simulink model "quad_control"  (Simulink 10.0)
settings: Solver=ode45  StartTime=0.0  StopTime=20  RelTol=1e-3  EnableMultiTasking=on
undefined symbols (not defined in the file): X, x, Y, Z
libraries: sm_lib x84, nesl_utility x46, simulink x30, fl_lib x4, sm_double_wishbone_suspension_lib x2, aerolibtransform2 x2, vrlib x1
(part 3 of 3)

== system quad_control/Controlled Quadrotor2/Quad and sensors/Quad_base_frame ==
  ReferenceFrame : sm_lib/Frames and  Transforms/Reference  Frame  BlockFunction=simmechanics.library.frames_transforms.reference_frame
      settings: SourceProductName=Simscape Multibody  SourceProductBaseCode=MS
  Solid : sm_lib/Body Elements/Solid  InertiaType=Custom  Mass=0.08666672774597016  MassUnits=kg  CenterOfMass=[0 0 0]  CenterOfMassUnits=cm  MomentsOfInertia=[2.1975971956009444 4.1375830610397539 2.1893109381556854]  MomentsOfInertiaUnits=kg*cm^2  ProductsOfInertia=[0 0 0]  ProductsOfInertiaUnits=kg*cm^2  DensityBased=on  Density=1000  DensityUnits=kg/(m^3)  GraphicType=FromGeometry  MarkerShape=Sphere  MarkerSize=10  MarkerSizeUnits=m  GraphicVisPropType=SimpleVisualProperties  GraphicDiffuseColor=[1.0 1.0 0.0]  GraphicSpecularColor=[0.5 0.5 0.5 1.0]  GraphicAmbientColor=[0.15 0.15 0.15 1.0]  GraphicEmissiveColor=[0.0 0.0 0.0 1.0]  GraphicShininess=75  GraphicOpacity=1  GeometryShape=FromFile  RectangleSize=[1 1]  RectangleSizeUnits=m  BrickDimensions=[1 1 1]  BrickDimensionUnits=m  CylinderRadius=1  CylinderRadiusUnits=m  CylinderLength=1  CylinderLengthUnits=m  SphereRadius=1  SphereRadiusUnits=m  EllipsoidRadii=[1 1 1]  EllipsoidRadiiUnits=m  ExtrusionCrossSection=[1 1; -1 1; -1 -1; 1 -1]  ExtrusionCrossSectionUnits=m  ExtrusionLength=1  ExtrusionLengthUnits=m  PolygonNumSides=3  PolygonOuterRadius=1  PolygonOuterRadiusUnits=m  ExtGeomFileType=STL  ExtGeomFileName=frame_motors_prt_Default_sldprt.STL  ExtGeomFileUnits=cm  RevolutionCrossSection=[1 1; 1 -1; 2 -1; 2 1]  RevolutionCrossSectionUnits=m  RevolutionExtent=Full  RevolutionAngle=180  RevolutionAngleUnits=deg  BlockFunction=simmechanics.library.body_elements.solid
  Transform : sm_lib/Frames and  Transforms/Rigid  Transform  TranslationMethod=Cartesian  TranslationLengthUnit=cm  TranslationStandardAxis=+Z  TranslationStandardOffset=0  TranslationCartesianOffset=[0.0025633413850464047 11.008725718944405 2.3329463666203418]  TranslationROffset=0  TranslationROffsetUnits=m  TranslationZOffset=0  TranslationZOffsetUnits=m  TranslationThetaOffset=0  TranslationThetaOffsetUnits=deg  RotationMethod=ArbitraryAxis  RotationAngleUnits=rad  RotationStandardAxis=+Z  RotationAngle=3.1415926535897896  RotationArbitraryAxis=[-1 -0 -0]  FollAlignAxisA=+X  BaseAlignAxisA=+Y  FollAlignAxisB=+Y  BaseAlignAxisB=+Z  RotationMatrix=[1 0 0; 0 1 0; 0 0 1]  BlockFunction=simmechanics.library.frames_transforms.rigid_transform
      settings: SourceProductName=Simscape Multibody  SourceProductBaseCode=MS
  Transform1 : sm_lib/Frames and  Transforms/Rigid  Transform  TranslationMethod=Cartesian  TranslationLengthUnit=cm  TranslationStandardAxis=+Z  TranslationStandardOffset=0  TranslationCartesianOffset=[0.002563341385239306 -10.791274281055713 2.3329463666202659]  TranslationROffset=0  TranslationROffsetUnits=m  TranslationZOffset=0  TranslationZOffsetUnits=m  TranslationThetaOffset=0  TranslationThetaOffsetUnits=deg  RotationMethod=ArbitraryAxis  RotationAngleUnits=rad  RotationStandardAxis=+Z  RotationAngle=3.1415926535897896  RotationArbitraryAxis=[-1 -0 -0]  FollAlignAxisA=+X  BaseAlignAxisA=+Y  FollAlignAxisB=+Y  BaseAlignAxisB=+Z  RotationMatrix=[1 0 0; 0 1 0; 0 0 1]  BlockFunction=simmechanics.library.frames_transforms.rigid_transform
      settings: SourceProductName=Simscape Multibody  SourceProductBaseCode=MS
  Transform2 : sm_lib/Frames and  Transforms/Rigid  Transform  TranslationMethod=Cartesian  TranslationLengthUnit=cm  TranslationStandardAxis=+Z  TranslationStandardOffset=0  TranslationCartesianOffset=[10.902563341385184 0.10872571894443728 2.3329463666203041]  TranslationROffset=0  TranslationROffsetUnits=m  TranslationZOffset=0  TranslationZOffsetUnits=m  TranslationThetaOffset=0  TranslationThetaOffsetUnits=deg  RotationMethod=ArbitraryAxis  RotationAngleUnits=rad  RotationStandardAxis=+Z  RotationAngle=3.1415926535897896  RotationArbitraryAxis=[-1 -0 -0]  FollAlignAxisA=+X  BaseAlignAxisA=+Y  FollAlignAxisB=+Y  BaseAlignAxisB=+Z  RotationMatrix=[1 0 0; 0 1 0; 0 0 1]  BlockFunction=simmechanics.library.frames_transforms.rigid_transform
      settings: SourceProductName=Simscape Multibody  SourceProductBaseCode=MS
  Transform3 : sm_lib/Frames and  Transforms/Rigid  Transform  TranslationMethod=Cartesian  TranslationLengthUnit=cm  TranslationStandardAxis=+Z  TranslationStandardOffset=0  TranslationCartesianOffset=[-10.897436658614925 0.10872571894425409 2.3329463666203041]  TranslationROffset=0  TranslationROffsetUnits=m  TranslationZOffset=0  TranslationZOffsetUnits=m  TranslationThetaOffset=0  TranslationThetaOffsetUnits=deg  RotationMethod=ArbitraryAxis  RotationAngleUnits=rad  RotationStandardAxis=+Z  RotationAngle=3.1415926535897896  RotationArbitraryAxis=[-1 -0 -0]  FollAlignAxisA=+X  BaseAlignAxisA=+Y  FollAlignAxisB=+Y  BaseAlignAxisB=+Z  RotationMatrix=[1 0 0; 0 1 0; 0 0 1]  BlockFunction=simmechanics.library.frames_transforms.rigid_transform
      settings: SourceProductName=Simscape Multibody  SourceProductBaseCode=MS
  F4 : PMIOPort  Side=Left
  F3 : PMIOPort  Port=2  Side=Right
  F2 : PMIOPort  Port=3  Side=Right
  F1 : PMIOPort  Port=4  Side=Right
  F : PMIOPort  Port=5  Side=Right
  connections:
  Transform3/LConn1 -- F4/RConn1 -- Transform/LConn1 -- Transform1/LConn1 -- Transform2/LConn1 -- ReferenceFrame/RConn1 -- Solid/RConn1
  Transform/RConn1 -- F/RConn1
  Transform1/RConn1 -- F1/RConn1
  Transform2/RConn1 -- F2/RConn1
  Transform3/RConn1 -- F3/RConn1

== system quad_control/Controlled Quadrotor2/world_base_and_floor/Floor ==
  ReferenceFrame : sm_lib/Frames and  Transforms/Reference  Frame  BlockFunction=simmechanics.library.frames_transforms.reference_frame
      settings: SourceProductName=Simscape Multibody  SourceProductBaseCode=MS
  Solid : sm_lib/Body Elements/Solid  InertiaType=Custom  Mass=3116.2499999999991  MassUnits=kg  CenterOfMass=[-7.9936057773011283e-16 -7.6605388699135795e-16 0.049999999999999996]  CenterOfMassUnits=m  MomentsOfInertia=[6494.7843749999947 6494.7843749999965 12984.374999999993]  MomentsOfInertiaUnits=kg*m^2  ProductsOfInertia=[0 0 -1.8451906669270059e-13]  ProductsOfInertiaUnits=kg*m^2  DensityBased=on  Density=1000  DensityUnits=kg/(m^3)  GraphicType=FromGeometry  MarkerShape=Sphere  MarkerSize=10  MarkerSizeUnits=m  GraphicVisPropType=SimpleVisualProperties  GraphicDiffuseColor=[0.0 0.4 0.4]  GraphicSpecularColor=[0.5 0.5 0.5 1.0]  GraphicAmbientColor=[0.15 0.15 0.15 1.0]  GraphicEmissiveColor=[0.0 0.0 0.0 1.0]  GraphicShininess=75  GraphicOpacity=1  GeometryShape=FromFile  RectangleSize=[1 1]  RectangleSizeUnits=m  BrickDimensions=[1 1 1]  BrickDimensionUnits=m  CylinderRadius=1  CylinderRadiusUnits=m  CylinderLength=1  CylinderLengthUnits=m  SphereRadius=1  SphereRadiusUnits=m  EllipsoidRadii=[1 1 1]  EllipsoidRadiiUnits=m  ExtrusionCrossSection=[1 1; -1 1; -1 -1; 1 -1]  ExtrusionCrossSectionUnits=m  ExtrusionLength=1  ExtrusionLengthUnits=m  PolygonNumSides=3  PolygonOuterRadius=1  PolygonOuterRadiusUnits=m  ExtGeomFileType=STL  ExtGeomFileName=floor_Default_sldprt.STL  ExtGeomFileUnits=m  RevolutionCrossSection=[1 1; 1 -1; 2 -1; 2 1]  RevolutionCrossSectionUnits=m  RevolutionExtent=Full  RevolutionAngle=180  RevolutionAngleUnits=deg  BlockFunction=simmechanics.library.body_elements.solid
  F : PMIOPort  Side=Left
  connections:
  ReferenceFrame/RConn1 -- Solid/RConn1 -- F/RConn1

== system quad_control/Controlled Quadrotor2/world_base_and_floor/floor2_1_RIGID ==
  ReferenceFrame : sm_lib/Frames and  Transforms/Reference  Frame  BlockFunction=simmechanics.library.frames_transforms.reference_frame
      settings: SourceProductName=Simscape Multibody  SourceProductBaseCode=MS
  Solid : sm_lib/Body Elements/Solid  InertiaType=Custom  Mass=2385.7763976055348  MassUnits=kg  CenterOfMass=[0.0012364446490796092 -0.0050570097364130108 0.050000002292491054]  CenterOfMassUnits=m  MomentsOfInertia=[5164.4159493771613 5045.1873132107048 10205.643458365917]  MomentsOfInertiaUnits=kg*m^2  ProductsOfInertia=[-1.8888660103894037e-06 -1.1052348010530633e-05 -9.5984261339922075]  ProductsOfInertiaUnits=kg*m^2  DensityBased=on  Density=1000  DensityUnits=kg/(m^3)  GraphicType=FromGeometry  MarkerShape=Sphere  MarkerSize=10  MarkerSizeUnits=m  GraphicVisPropType=SimpleVisualProperties  GraphicDiffuseColor=[1 1 1]  GraphicSpecularColor=[0.5 0.5 0.5 1.0]  GraphicAmbientColor=[0.15 0.15 0.15 1.0]  GraphicEmissiveColor=[0.0 0.0 0.0 1.0]  GraphicShininess=75  GraphicOpacity=1  GeometryShape=FromFile  RectangleSize=[1 1]  RectangleSizeUnits=m  BrickDimensions=[1 1 1]  BrickDimensionUnits=m  CylinderRadius=1  CylinderRadiusUnits=m  CylinderLength=1  CylinderLengthUnits=m  SphereRadius=1  SphereRadiusUnits=m  EllipsoidRadii=[1 1 1]  EllipsoidRadiiUnits=m  ExtrusionCrossSection=[1 1; -1 1; -1 -1; 1 -1]  ExtrusionCrossSectionUnits=m  ExtrusionLength=1  ExtrusionLengthUnits=m  PolygonNumSides=3  PolygonOuterRadius=1  PolygonOuterRadiusUnits=m  ExtGeomFileType=STL  ExtGeomFileName=floor2_Default_sldprt.STL  ExtGeomFileUnits=m  RevolutionCrossSection=[1 1; 1 -1; 2 -1; 2 1]  RevolutionCrossSectionUnits=m  RevolutionExtent=Full  RevolutionAngle=180  RevolutionAngleUnits=deg  BlockFunction=simmechanics.library.body_elements.solid
  Transform : sm_lib/Frames and  Transforms/Rigid  Transform  TranslationMethod=Cartesian  TranslationLengthUnit=m  TranslationStandardAxis=+Z  TranslationStandardOffset=0  TranslationCartesianOffset=[0 0 0.099999999999999978]  TranslationROffset=0  TranslationROffsetUnits=m  TranslationZOffset=0  TranslationZOffsetUnits=m  TranslationThetaOffset=0  TranslationThetaOffsetUnits=deg  RotationMethod=ArbitraryAxis  RotationAngleUnits=rad  RotationStandardAxis=+Z  RotationAngle=0  RotationArbitraryAxis=[0 0 0]  FollAlignAxisA=+X  BaseAlignAxisA=+Y  FollAlignAxisB=+Y  BaseAlignAxisB=+Z  RotationMatrix=[1 0 0; 0 1 0; 0 0 1]  BlockFunction=simmechanics.library.frames_transforms.rigid_transform
      settings: SourceProductName=Simscape Multibody  SourceProductBaseCode=MS
  F1 : PMIOPort  Side=Left
  connections:
  ReferenceFrame/RConn1 -- Solid/RConn1 -- Transform/LConn1 -- F1/RConn1

== system quad_control/Controlled Quadrotor2/world_base_and_floor/text2_1_RIGID ==
  ReferenceFrame : sm_lib/Frames and  Transforms/Reference  Frame  BlockFunction=simmechanics.library.frames_transforms.reference_frame
      settings: SourceProductName=Simscape Multibody  SourceProductBaseCode=MS
  Solid : sm_lib/Body Elements/Solid  InertiaType=Custom  Mass=52.995915434963941  MassUnits=kg  CenterOfMass=[0.014313236427579184 0.013266517593960889 0.050000099576434989]  CenterOfMassUnits=m  MomentsOfInertia=[1.2121218611867071 89.98262862045047 91.106423651417629]  MomentsOfInertiaUnits=kg*m^2  ProductsOfInertia=[-2.6542355925642964e-07 -7.9011888790530038e-06 1.0815100741629544]  ProductsOfInertiaUnits=kg*m^2  DensityBased=on  Density=1000  DensityUnits=kg/(m^3)  GraphicType=FromGeometry  MarkerShape=Sphere  MarkerSize=10  MarkerSizeUnits=m  GraphicVisPropType=SimpleVisualProperties  GraphicDiffuseColor=[1.0 1.0 0.4]  GraphicSpecularColor=[0.5 0.5 0.5 1.0]  GraphicAmbientColor=[0.15 0.15 0.15 1.0]  GraphicEmissiveColor=[0.0 0.0 0.0 1.0]  GraphicShininess=75  GraphicOpacity=1  GeometryShape=FromFile  RectangleSize=[1 1]  RectangleSizeUnits=m  BrickDimensions=[1 1 1]  BrickDimensionUnits=m  CylinderRadius=1  CylinderRadiusUnits=m  CylinderLength=1  CylinderLengthUnits=m  SphereRadius=1  SphereRadiusUnits=m  EllipsoidRadii=[1 1 1]  EllipsoidRadiiUnits=m  ExtrusionCrossSection=[1 1; -1 1; -1 -1; 1 -1]  ExtrusionCrossSectionUnits=m  ExtrusionLength=1  ExtrusionLengthUnits=m  PolygonNumSides=3  PolygonOuterRadius=1  PolygonOuterRadiusUnits=m  ExtGeomFileType=STL  ExtGeomFileName=text2_Default_sldprt.STL  ExtGeomFileUnits=m  RevolutionCrossSection=[1 1; 1 -1; 2 -1; 2 1]  RevolutionCrossSectionUnits=m  RevolutionExtent=Full  RevolutionAngle=180  RevolutionAngleUnits=deg  BlockFunction=simmechanics.library.body_elements.solid
  Transform : sm_lib/Frames and  Transforms/Rigid  Transform  TranslationMethod=Cartesian  TranslationLengthUnit=m  TranslationStandardAxis=+Z  TranslationStandardOffset=0  TranslationCartesianOffset=[-0.0410033698434355 2.1287464318513987 -1.3877787807814457e-17]  TranslationROffset=0  TranslationROffsetUnits=m  TranslationZOffset=0  TranslationZOffsetUnits=m  TranslationThetaOffset=0  TranslationThetaOffsetUnits=deg  RotationMethod=ArbitraryAxis  RotationAngleUnits=rad  RotationStandardAxis=+Z  RotationAngle=0  RotationArbitraryAxis=[0 0 0]  FollAlignAxisA=+X  BaseAlignAxisA=+Y  FollAlignAxisB=+Y  BaseAlignAxisB=+Z  RotationMatrix=[1 0 0; 0 1 0; 0 0 1]  BlockFunction=simmechanics.library.frames_transforms.rigid_transform
      settings: SourceProductName=Simscape Multibody  SourceProductBaseCode=MS
  F1 : PMIOPort  Side=Left
  connections:
  Transform/LConn1 -- F1/RConn1 -- ReferenceFrame/RConn1 -- Solid/RConn1

== system quad_control/Controlled Quadrotor1/Quad and sensors/Engine1/x5x3R_Propeller_1_RIGID ==
  ReferenceFrame : sm_lib/Frames and  Transforms/Reference  Frame  BlockFunction=simmechanics.library.frames_transforms.reference_frame
      settings: SourceProductName=Simscape Multibody  SourceProductBaseCode=MS
  Solid : sm_lib/Body Elements/Solid  InertiaType=Custom  Mass=0.0016554437499046806  MassUnits=kg  CenterOfMass=[-9.4091969973109005e-06 1.1743794416735667 -1.1742585501049463]  CenterOfMassUnits=mm  MomentsOfInertia=[1.470390252449407 0.013647828129438603 1.4797649971234468]  MomentsOfInertiaUnits=kg*mm^2  ProductsOfInertia=[7.6225900321173699e-07 3.0379766986994385e-08 -0.023426386413677357]  ProductsOfInertiaUnits=kg*mm^2  DensityBased=on  Density=1000  DensityUnits=kg/(m^3)  GraphicType=FromGeometry  MarkerShape=Sphere  MarkerSize=10  MarkerSizeUnits=m  GraphicVisPropType=SimpleVisualProperties  GraphicDiffuseColor=[1.0 0.2 0.0]  GraphicSpecularColor=[0.5 0.5 0.5 1.0]  GraphicAmbientColor=[0.15 0.15 0.15 1.0]  GraphicEmissiveColor=[0.0 0.0 0.0 1.0]  GraphicShininess=75  GraphicOpacity=1  GeometryShape=FromFile  RectangleSize=[1 1]  RectangleSizeUnits=m  BrickDimensions=[1 1 1]  BrickDimensionUnits=m  CylinderRadius=1  CylinderRadiusUnits=m  CylinderLength=1  CylinderLengthUnits=m  SphereRadius=1  SphereRadiusUnits=m  EllipsoidRadii=[1 1 1]  EllipsoidRadiiUnits=m  ExtrusionCrossSection=[1 1; -1 1; -1 -1; 1 -1]  ExtrusionCrossSectionUnits=m  ExtrusionLength=1  ExtrusionLengthUnits=m  PolygonNumSides=3  PolygonOuterRadius=1  PolygonOuterRadiusUnits=m  ExtGeomFileType=STL  ExtGeomFileName=5x3R Propeller_Default_sldprt.STL  ExtGeomFileUnits=mm  RevolutionCrossSection=[1 1; 1 -1; 2 -1; 2 1]  RevolutionCrossSectionUnits=m  RevolutionExtent=Full  RevolutionAngle=180  RevolutionAngleUnits=deg  BlockFunction=simmechanics.library.body_elements.solid
  Transform : sm_lib/Frames and  Transforms/Rigid  Transform  TranslationMethod=Cartesian  TranslationLengthUnit=cm  TranslationStandardAxis=+Z  TranslationStandardOffset=0  TranslationCartesianOffset=[2.2204460492503131e-16 0.117384178389595 0.70211061015740817]  TranslationROffset=0  TranslationROffsetUnits=m  TranslationZOffset=0  TranslationZOffsetUnits=m  TranslationThetaOffset=0  TranslationThetaOffsetUnits=deg  RotationMethod=ArbitraryAxis  RotationAngleUnits=rad  RotationStandardAxis=+Z  RotationAngle=3.14159265358979  RotationArbitraryAxis=[-1 -2.9659662640582496e-31 1.7826123921481009e-16]  FollAlignAxisA=+X  BaseAlignAxisA=+Y  FollAlignAxisB=+Y  BaseAlignAxisB=+Z  RotationMatrix=[1 0 0; 0 1 0; 0 0 1]  BlockFunction=simmechanics.library.frames_transforms.rigid_transform
      settings: SourceProductName=Simscape Multibody  SourceProductBaseCode=MS
  F : PMIOPort  Side=Left
  connections:
  ReferenceFrame/RConn1 -- Solid/RConn1 -- Transform/LConn1
  Transform/RConn1 -- F/RConn1

== system quad_control/Controlled Quadrotor1/Quad and sensors/Engine2/x5x3L_Propeller_1_RIGID ==
  ReferenceFrame : sm_lib/Frames and  Transforms/Reference  Frame  BlockFunction=simmechanics.library.frames_transforms.reference_frame
      settings: SourceProductName=Simscape Multibody  SourceProductBaseCode=MS
  Solid : sm_lib/Body Elements/Solid  InertiaType=Custom  Mass=0.0016554447827057072  MassUnits=kg  CenterOfMass=[-1.7940684369643517e-05 0.00054453975800766252 -0.0036928877456850299]  CenterOfMassUnits=mm  MomentsOfInertia=[1.4703904309245746 0.013647735813102926 1.4797650826066844]  MomentsOfInertiaUnits=kg*mm^2  ProductsOfInertia=[7.6907097391567737e-07 1.5969591997949786e-08 -0.023426501249338923]  ProductsOfInertiaUnits=kg*mm^2  DensityBased=on  Density=1000  DensityUnits=kg/(m^3)  GraphicType=FromGeometry  MarkerShape=Sphere  MarkerSize=10  MarkerSizeUnits=m  GraphicVisPropType=SimpleVisualProperties  GraphicDiffuseColor=[0.0 0.0 0.0]  GraphicSpecularColor=[0.5 0.5 0.5 1.0]  GraphicAmbientColor=[0.15 0.15 0.15 1.0]  GraphicEmissiveColor=[0.0 0.0 0.0 1.0]  GraphicShininess=75  GraphicOpacity=1  GeometryShape=FromFile  RectangleSize=[1 1]  RectangleSizeUnits=m  BrickDimensions=[1 1 1]  BrickDimensionUnits=m  CylinderRadius=1  CylinderRadiusUnits=m  CylinderLength=1  CylinderLengthUnits=m  SphereRadius=1  SphereRadiusUnits=m  EllipsoidRadii=[1 1 1]  EllipsoidRadiiUnits=m  ExtrusionCrossSection=[1 1; -1 1; -1 -1; 1 -1]  ExtrusionCrossSectionUnits=m  ExtrusionLength=1  ExtrusionLengthUnits=m  PolygonNumSides=3  PolygonOuterRadius=1  PolygonOuterRadiusUnits=m  ExtGeomFileType=STL  ExtGeomFileName=5x3L Propeller_Default_sldprt.STL  ExtGeomFileUnits=mm  RevolutionCrossSection=[1 1; 1 -1; 2 -1; 2 1]  RevolutionCrossSectionUnits=m  RevolutionExtent=Full  RevolutionAngle=180  RevolutionAngleUnits=deg  BlockFunction=simmechanics.library.body_elements.solid
  Transform : sm_lib/Frames and  Transforms/Rigid  Transform  TranslationMethod=Cartesian  TranslationLengthUnit=cm  TranslationStandardAxis=+Z  TranslationStandardOffset=0  TranslationCartesianOffset=[-8.1659826880039994e-17 -5.3402587403471918e-15 0.81916743857986374]  TranslationROffset=0  TranslationROffsetUnits=m  TranslationZOffset=0  TranslationZOffsetUnits=m  TranslationThetaOffset=0  TranslationThetaOffsetUnits=deg  RotationMethod=ArbitraryAxis  RotationAngleUnits=rad  RotationStandardAxis=+Z  RotationAngle=3.1415926535897896  RotationArbitraryAxis=[-1 3.3672490814660118e-32 -1.9301742002667719e-17]  FollAlignAxisA=+X  BaseAlignAxisA=+Y  FollAlignAxisB=+Y  BaseAlignAxisB=+Z  RotationMatrix=[1 0 0; 0 1 0; 0 0 1]  BlockFunction=simmechanics.library.frames_transforms.rigid_transform
      settings: SourceProductName=Simscape Multibody  SourceProductBaseCode=MS
  F : PMIOPort  Side=Left
  connections:
  ReferenceFrame/RConn1 -- Solid/RConn1 -- Transform/LConn1
  Transform/RConn1 -- F/RConn1

== system quad_control/Controlled Quadrotor1/Quad and sensors/Engine3/x5x3R_Propeller_2_RIGID ==
  ReferenceFrame : sm_lib/Frames and  Transforms/Reference  Frame  BlockFunction=simmechanics.library.frames_transforms.reference_frame
      settings: SourceProductName=Simscape Multibody  SourceProductBaseCode=MS
  Solid : sm_lib/Body Elements/Solid  InertiaType=Custom  Mass=0.0016554437499046806  MassUnits=kg  CenterOfMass=[-9.4091969973109005e-06 1.1743794416735667 -1.1742585501049463]  CenterOfMassUnits=mm  MomentsOfInertia=[1.470390252449407 0.013647828129438603 1.4797649971234468]  MomentsOfInertiaUnits=kg*mm^2  ProductsOfInertia=[7.6225900321173699e-07 3.0379766986994385e-08 -0.023426386413677357]  ProductsOfInertiaUnits=kg*mm^2  DensityBased=on  Density=1000  DensityUnits=kg/(m^3)  GraphicType=FromGeometry  MarkerShape=Sphere  MarkerSize=10  MarkerSizeUnits=m  GraphicVisPropType=SimpleVisualProperties  GraphicDiffuseColor=[0.0 0.0 0.0]  GraphicSpecularColor=[0.5 0.5 0.5 1.0]  GraphicAmbientColor=[0.15 0.15 0.15 1.0]  GraphicEmissiveColor=[0.0 0.0 0.0 1.0]  GraphicShininess=75  GraphicOpacity=1  GeometryShape=FromFile  RectangleSize=[1 1]  RectangleSizeUnits=m  BrickDimensions=[1 1 1]  BrickDimensionUnits=m  CylinderRadius=1  CylinderRadiusUnits=m  CylinderLength=1  CylinderLengthUnits=m  SphereRadius=1  SphereRadiusUnits=m  EllipsoidRadii=[1 1 1]  EllipsoidRadiiUnits=m  ExtrusionCrossSection=[1 1; -1 1; -1 -1; 1 -1]  ExtrusionCrossSectionUnits=m  ExtrusionLength=1  ExtrusionLengthUnits=m  PolygonNumSides=3  PolygonOuterRadius=1  PolygonOuterRadiusUnits=m  ExtGeomFileType=STL  ExtGeomFileName=5x3R Propeller_Default_sldprt.STL  ExtGeomFileUnits=mm  RevolutionCrossSection=[1 1; 1 -1; 2 -1; 2 1]  RevolutionCrossSectionUnits=m  RevolutionExtent=Full  RevolutionAngle=180  RevolutionAngleUnits=deg  BlockFunction=simmechanics.library.body_elements.solid
  Transform : sm_lib/Frames and  Transforms/Rigid  Transform  TranslationMethod=Cartesian  TranslationLengthUnit=cm  TranslationStandardAxis=+Z  TranslationStandardOffset=0  TranslationCartesianOffset=[-9.721390359374027e-15 0.11738417838958951 0.70211061015740495]  TranslationROffset=0  TranslationROffsetUnits=m  TranslationZOffset=0  TranslationZOffsetUnits=m  TranslationThetaOffset=0  TranslationThetaOffsetUnits=deg  RotationMethod=ArbitraryAxis  RotationAngleUnits=rad  RotationStandardAxis=+Z  RotationAngle=3.14159265358979  RotationArbitraryAxis=[-1 -6.9195844784490633e-32 4.2800760370596708e-17]  FollAlignAxisA=+X  BaseAlignAxisA=+Y  FollAlignAxisB=+Y  BaseAlignAxisB=+Z  RotationMatrix=[1 0 0; 0 1 0; 0 0 1]  BlockFunction=simmechanics.library.frames_transforms.rigid_transform
      settings: SourceProductName=Simscape Multibody  SourceProductBaseCode=MS
  F : PMIOPort  Side=Left
  connections:
  ReferenceFrame/RConn1 -- Solid/RConn1 -- Transform/LConn1
  Transform/RConn1 -- F/RConn1

== system quad_control/Controlled Quadrotor1/Quad and sensors/Engine4/x5x3L_Propeller_2_RIGID ==
  ReferenceFrame : sm_lib/Frames and  Transforms/Reference  Frame  BlockFunction=simmechanics.library.frames_transforms.reference_frame
      settings: SourceProductName=Simscape Multibody  SourceProductBaseCode=MS
  Solid : sm_lib/Body Elements/Solid  InertiaType=Custom  Mass=0.0016554447827057072  MassUnits=kg  CenterOfMass=[-1.7940684369643517e-05 0.00054453975800766252 -0.0036928877456850299]  CenterOfMassUnits=mm  MomentsOfInertia=[1.4703904309245746 0.013647735813102926 1.4797650826066844]  MomentsOfInertiaUnits=kg*mm^2  ProductsOfInertia=[7.6907097391567737e-07 1.5969591997949786e-08 -0.023426501249338923]  ProductsOfInertiaUnits=kg*mm^2  DensityBased=on  Density=1000  DensityUnits=kg/(m^3)  GraphicType=FromGeometry  MarkerShape=Sphere  MarkerSize=10  MarkerSizeUnits=m  GraphicVisPropType=SimpleVisualProperties  GraphicDiffuseColor=[0.0 0.0 0.0]  GraphicSpecularColor=[0.5 0.5 0.5 1.0]  GraphicAmbientColor=[0.15 0.15 0.15 1.0]  GraphicEmissiveColor=[0.0 0.0 0.0 1.0]  GraphicShininess=75  GraphicOpacity=1  GeometryShape=FromFile  RectangleSize=[1 1]  RectangleSizeUnits=m  BrickDimensions=[1 1 1]  BrickDimensionUnits=m  CylinderRadius=1  CylinderRadiusUnits=m  CylinderLength=1  CylinderLengthUnits=m  SphereRadius=1  SphereRadiusUnits=m  EllipsoidRadii=[1 1 1]  EllipsoidRadiiUnits=m  ExtrusionCrossSection=[1 1; -1 1; -1 -1; 1 -1]  ExtrusionCrossSectionUnits=m  ExtrusionLength=1  ExtrusionLengthUnits=m  PolygonNumSides=3  PolygonOuterRadius=1  PolygonOuterRadiusUnits=m  ExtGeomFileType=STL  ExtGeomFileName=5x3L Propeller_Default_sldprt.STL  ExtGeomFileUnits=mm  RevolutionCrossSection=[1 1; 1 -1; 2 -1; 2 1]  RevolutionCrossSectionUnits=m  RevolutionExtent=Full  RevolutionAngle=180  RevolutionAngleUnits=deg  BlockFunction=simmechanics.library.body_elements.solid
  Transform : sm_lib/Frames and  Transforms/Rigid  Transform  TranslationMethod=Cartesian  TranslationLengthUnit=cm  TranslationStandardAxis=+Z  TranslationStandardOffset=0  TranslationCartesianOffset=[1.1902527643660046e-20 -5.3306783429948579e-15 0.8191674385798644]  TranslationROffset=0  TranslationROffsetUnits=m  TranslationZOffset=0  TranslationZOffsetUnits=m  TranslationThetaOffset=0  TranslationThetaOffsetUnits=deg  RotationMethod=ArbitraryAxis  RotationAngleUnits=rad  RotationStandardAxis=+Z  RotationAngle=3.1415926535897896  RotationArbitraryAxis=[-1 5.1433426364519453e-33 -2.9461315815038046e-18]  FollAlignAxisA=+X  BaseAlignAxisA=+Y  FollAlignAxisB=+Y  BaseAlignAxisB=+Z  RotationMatrix=[1 0 0; 0 1 0; 0 0 1]  BlockFunction=simmechanics.library.frames_transforms.rigid_transform
      settings: SourceProductName=Simscape Multibody  SourceProductBaseCode=MS
  F : PMIOPort  Side=Left
  connections:
  ReferenceFrame/RConn1 -- Solid/RConn1 -- Transform/LConn1
  Transform/RConn1 -- F/RConn1

== system quad_control/Controlled Quadrotor2/Quad and sensors/Engine1/x5x3R_Propeller_1_RIGID ==
  ReferenceFrame : sm_lib/Frames and  Transforms/Reference  Frame  BlockFunction=simmechanics.library.frames_transforms.reference_frame
      settings: SourceProductName=Simscape Multibody  SourceProductBaseCode=MS
  Solid : sm_lib/Body Elements/Solid  InertiaType=Custom  Mass=0.0016554437499046806  MassUnits=kg  CenterOfMass=[-9.4091969973109005e-06 1.1743794416735667 -1.1742585501049463]  CenterOfMassUnits=mm  MomentsOfInertia=[1.470390252449407 0.013647828129438603 1.4797649971234468]  MomentsOfInertiaUnits=kg*mm^2  ProductsOfInertia=[7.6225900321173699e-07 3.0379766986994385e-08 -0.023426386413677357]  ProductsOfInertiaUnits=kg*mm^2  DensityBased=on  Density=1000  DensityUnits=kg/(m^3)  GraphicType=FromGeometry  MarkerShape=Sphere  MarkerSize=10  MarkerSizeUnits=m  GraphicVisPropType=SimpleVisualProperties  GraphicDiffuseColor=[1.0 0.2 0.0]  GraphicSpecularColor=[0.5 0.5 0.5 1.0]  GraphicAmbientColor=[0.15 0.15 0.15 1.0]  GraphicEmissiveColor=[0.0 0.0 0.0 1.0]  GraphicShininess=75  GraphicOpacity=1  GeometryShape=FromFile  RectangleSize=[1 1]  RectangleSizeUnits=m  BrickDimensions=[1 1 1]  BrickDimensionUnits=m  CylinderRadius=1  CylinderRadiusUnits=m  CylinderLength=1  CylinderLengthUnits=m  SphereRadius=1  SphereRadiusUnits=m  EllipsoidRadii=[1 1 1]  EllipsoidRadiiUnits=m  ExtrusionCrossSection=[1 1; -1 1; -1 -1; 1 -1]  ExtrusionCrossSectionUnits=m  ExtrusionLength=1  ExtrusionLengthUnits=m  PolygonNumSides=3  PolygonOuterRadius=1  PolygonOuterRadiusUnits=m  ExtGeomFileType=STL  ExtGeomFileName=5x3R Propeller_Default_sldprt.STL  ExtGeomFileUnits=mm  RevolutionCrossSection=[1 1; 1 -1; 2 -1; 2 1]  RevolutionCrossSectionUnits=m  RevolutionExtent=Full  RevolutionAngle=180  RevolutionAngleUnits=deg  BlockFunction=simmechanics.library.body_elements.solid
  Transform : sm_lib/Frames and  Transforms/Rigid  Transform  TranslationMethod=Cartesian  TranslationLengthUnit=cm  TranslationStandardAxis=+Z  TranslationStandardOffset=0  TranslationCartesianOffset=[2.2204460492503131e-16 0.117384178389595 0.70211061015740817]  TranslationROffset=0  TranslationROffsetUnits=m  TranslationZOffset=0  TranslationZOffsetUnits=m  TranslationThetaOffset=0  TranslationThetaOffsetUnits=deg  RotationMethod=ArbitraryAxis  RotationAngleUnits=rad  RotationStandardAxis=+Z  RotationAngle=3.14159265358979  RotationArbitraryAxis=[-1 -2.9659662640582496e-31 1.7826123921481009e-16]  FollAlignAxisA=+X  BaseAlignAxisA=+Y  FollAlignAxisB=+Y  BaseAlignAxisB=+Z  RotationMatrix=[1 0 0; 0 1 0; 0 0 1]  BlockFunction=simmechanics.library.frames_transforms.rigid_transform
      settings: SourceProductName=Simscape Multibody  SourceProductBaseCode=MS
  F : PMIOPort  Side=Left
  connections:
  ReferenceFrame/RConn1 -- Solid/RConn1 -- Transform/LConn1
  Transform/RConn1 -- F/RConn1

== system quad_control/Controlled Quadrotor2/Quad and sensors/Engine2/x5x3L_Propeller_1_RIGID ==
  ReferenceFrame : sm_lib/Frames and  Transforms/Reference  Frame  BlockFunction=simmechanics.library.frames_transforms.reference_frame
      settings: SourceProductName=Simscape Multibody  SourceProductBaseCode=MS
  Solid : sm_lib/Body Elements/Solid  InertiaType=Custom  Mass=0.0016554447827057072  MassUnits=kg  CenterOfMass=[-1.7940684369643517e-05 0.00054453975800766252 -0.0036928877456850299]  CenterOfMassUnits=mm  MomentsOfInertia=[1.4703904309245746 0.013647735813102926 1.4797650826066844]  MomentsOfInertiaUnits=kg*mm^2  ProductsOfInertia=[7.6907097391567737e-07 1.5969591997949786e-08 -0.023426501249338923]  ProductsOfInertiaUnits=kg*mm^2  DensityBased=on  Density=1000  DensityUnits=kg/(m^3)  GraphicType=FromGeometry  MarkerShape=Sphere  MarkerSize=10  MarkerSizeUnits=m  GraphicVisPropType=SimpleVisualProperties  GraphicDiffuseColor=[0.0 0.0 0.0]  GraphicSpecularColor=[0.5 0.5 0.5 1.0]  GraphicAmbientColor=[0.15 0.15 0.15 1.0]  GraphicEmissiveColor=[0.0 0.0 0.0 1.0]  GraphicShininess=75  GraphicOpacity=1  GeometryShape=FromFile  RectangleSize=[1 1]  RectangleSizeUnits=m  BrickDimensions=[1 1 1]  BrickDimensionUnits=m  CylinderRadius=1  CylinderRadiusUnits=m  CylinderLength=1  CylinderLengthUnits=m  SphereRadius=1  SphereRadiusUnits=m  EllipsoidRadii=[1 1 1]  EllipsoidRadiiUnits=m  ExtrusionCrossSection=[1 1; -1 1; -1 -1; 1 -1]  ExtrusionCrossSectionUnits=m  ExtrusionLength=1  ExtrusionLengthUnits=m  PolygonNumSides=3  PolygonOuterRadius=1  PolygonOuterRadiusUnits=m  ExtGeomFileType=STL  ExtGeomFileName=5x3L Propeller_Default_sldprt.STL  ExtGeomFileUnits=mm  RevolutionCrossSection=[1 1; 1 -1; 2 -1; 2 1]  RevolutionCrossSectionUnits=m  RevolutionExtent=Full  RevolutionAngle=180  RevolutionAngleUnits=deg  BlockFunction=simmechanics.library.body_elements.solid
  Transform : sm_lib/Frames and  Transforms/Rigid  Transform  TranslationMethod=Cartesian  TranslationLengthUnit=cm  TranslationStandardAxis=+Z  TranslationStandardOffset=0  TranslationCartesianOffset=[-8.1659826880039994e-17 -5.3402587403471918e-15 0.81916743857986374]  TranslationROffset=0  TranslationROffsetUnits=m  TranslationZOffset=0  TranslationZOffsetUnits=m  TranslationThetaOffset=0  TranslationThetaOffsetUnits=deg  RotationMethod=ArbitraryAxis  RotationAngleUnits=rad  RotationStandardAxis=+Z  RotationAngle=3.1415926535897896  RotationArbitraryAxis=[-1 3.3672490814660118e-32 -1.9301742002667719e-17]  FollAlignAxisA=+X  BaseAlignAxisA=+Y  FollAlignAxisB=+Y  BaseAlignAxisB=+Z  RotationMatrix=[1 0 0; 0 1 0; 0 0 1]  BlockFunction=simmechanics.library.frames_transforms.rigid_transform
      settings: SourceProductName=Simscape Multibody  SourceProductBaseCode=MS
  F : PMIOPort  Side=Left
  connections:
  ReferenceFrame/RConn1 -- Solid/RConn1 -- Transform/LConn1
  Transform/RConn1 -- F/RConn1

== system quad_control/Controlled Quadrotor2/Quad and sensors/Engine3/x5x3R_Propeller_2_RIGID ==
  ReferenceFrame : sm_lib/Frames and  Transforms/Reference  Frame  BlockFunction=simmechanics.library.frames_transforms.reference_frame
      settings: SourceProductName=Simscape Multibody  SourceProductBaseCode=MS
  Solid : sm_lib/Body Elements/Solid  InertiaType=Custom  Mass=0.0016554437499046806  MassUnits=kg  CenterOfMass=[-9.4091969973109005e-06 1.1743794416735667 -1.1742585501049463]  CenterOfMassUnits=mm  MomentsOfInertia=[1.470390252449407 0.013647828129438603 1.4797649971234468]  MomentsOfInertiaUnits=kg*mm^2  ProductsOfInertia=[7.6225900321173699e-07 3.0379766986994385e-08 -0.023426386413677357]  ProductsOfInertiaUnits=kg*mm^2  DensityBased=on  Density=1000  DensityUnits=kg/(m^3)  GraphicType=FromGeometry  MarkerShape=Sphere  MarkerSize=10  MarkerSizeUnits=m  GraphicVisPropType=SimpleVisualProperties  GraphicDiffuseColor=[0.0 0.0 0.0]  GraphicSpecularColor=[0.5 0.5 0.5 1.0]  GraphicAmbientColor=[0.15 0.15 0.15 1.0]  GraphicEmissiveColor=[0.0 0.0 0.0 1.0]  GraphicShininess=75  GraphicOpacity=1  GeometryShape=FromFile  RectangleSize=[1 1]  RectangleSizeUnits=m  BrickDimensions=[1 1 1]  BrickDimensionUnits=m  CylinderRadius=1  CylinderRadiusUnits=m  CylinderLength=1  CylinderLengthUnits=m  SphereRadius=1  SphereRadiusUnits=m  EllipsoidRadii=[1 1 1]  EllipsoidRadiiUnits=m  ExtrusionCrossSection=[1 1; -1 1; -1 -1; 1 -1]  ExtrusionCrossSectionUnits=m  ExtrusionLength=1  ExtrusionLengthUnits=m  PolygonNumSides=3  PolygonOuterRadius=1  PolygonOuterRadiusUnits=m  ExtGeomFileType=STL  ExtGeomFileName=5x3R Propeller_Default_sldprt.STL  ExtGeomFileUnits=mm  RevolutionCrossSection=[1 1; 1 -1; 2 -1; 2 1]  RevolutionCrossSectionUnits=m  RevolutionExtent=Full  RevolutionAngle=180  RevolutionAngleUnits=deg  BlockFunction=simmechanics.library.body_elements.solid
  Transform : sm_lib/Frames and  Transforms/Rigid  Transform  TranslationMethod=Cartesian  TranslationLengthUnit=cm  TranslationStandardAxis=+Z  TranslationStandardOffset=0  TranslationCartesianOffset=[-9.721390359374027e-15 0.11738417838958951 0.70211061015740495]  TranslationROffset=0  TranslationROffsetUnits=m  TranslationZOffset=0  TranslationZOffsetUnits=m  TranslationThetaOffset=0  TranslationThetaOffsetUnits=deg  RotationMethod=ArbitraryAxis  RotationAngleUnits=rad  RotationStandardAxis=+Z  RotationAngle=3.14159265358979  RotationArbitraryAxis=[-1 -6.9195844784490633e-32 4.2800760370596708e-17]  FollAlignAxisA=+X  BaseAlignAxisA=+Y  FollAlignAxisB=+Y  BaseAlignAxisB=+Z  RotationMatrix=[1 0 0; 0 1 0; 0 0 1]  BlockFunction=simmechanics.library.frames_transforms.rigid_transform
      settings: SourceProductName=Simscape Multibody  SourceProductBaseCode=MS
  F : PMIOPort  Side=Left
  connections:
  ReferenceFrame/RConn1 -- Solid/RConn1 -- Transform/LConn1
  Transform/RConn1 -- F/RConn1

== system quad_control/Controlled Quadrotor2/Quad and sensors/Engine4/x5x3L_Propeller_2_RIGID ==
  ReferenceFrame : sm_lib/Frames and  Transforms/Reference  Frame  BlockFunction=simmechanics.library.frames_transforms.reference_frame
      settings: SourceProductName=Simscape Multibody  SourceProductBaseCode=MS
  Solid : sm_lib/Body Elements/Solid  InertiaType=Custom  Mass=0.0016554447827057072  MassUnits=kg  CenterOfMass=[-1.7940684369643517e-05 0.00054453975800766252 -0.0036928877456850299]  CenterOfMassUnits=mm  MomentsOfInertia=[1.4703904309245746 0.013647735813102926 1.4797650826066844]  MomentsOfInertiaUnits=kg*mm^2  ProductsOfInertia=[7.6907097391567737e-07 1.5969591997949786e-08 -0.023426501249338923]  ProductsOfInertiaUnits=kg*mm^2  DensityBased=on  Density=1000  DensityUnits=kg/(m^3)  GraphicType=FromGeometry  MarkerShape=Sphere  MarkerSize=10  MarkerSizeUnits=m  GraphicVisPropType=SimpleVisualProperties  GraphicDiffuseColor=[0.0 0.0 0.0]  GraphicSpecularColor=[0.5 0.5 0.5 1.0]  GraphicAmbientColor=[0.15 0.15 0.15 1.0]  GraphicEmissiveColor=[0.0 0.0 0.0 1.0]  GraphicShininess=75  GraphicOpacity=1  GeometryShape=FromFile  RectangleSize=[1 1]  RectangleSizeUnits=m  BrickDimensions=[1 1 1]  BrickDimensionUnits=m  CylinderRadius=1  CylinderRadiusUnits=m  CylinderLength=1  CylinderLengthUnits=m  SphereRadius=1  SphereRadiusUnits=m  EllipsoidRadii=[1 1 1]  EllipsoidRadiiUnits=m  ExtrusionCrossSection=[1 1; -1 1; -1 -1; 1 -1]  ExtrusionCrossSectionUnits=m  ExtrusionLength=1  ExtrusionLengthUnits=m  PolygonNumSides=3  PolygonOuterRadius=1  PolygonOuterRadiusUnits=m  ExtGeomFileType=STL  ExtGeomFileName=5x3L Propeller_Default_sldprt.STL  ExtGeomFileUnits=mm  RevolutionCrossSection=[1 1; 1 -1; 2 -1; 2 1]  RevolutionCrossSectionUnits=m  RevolutionExtent=Full  RevolutionAngle=180  RevolutionAngleUnits=deg  BlockFunction=simmechanics.library.body_elements.solid
  Transform : sm_lib/Frames and  Transforms/Rigid  Transform  TranslationMethod=Cartesian  TranslationLengthUnit=cm  TranslationStandardAxis=+Z  TranslationStandardOffset=0  TranslationCartesianOffset=[1.1902527643660046e-20 -5.3306783429948579e-15 0.8191674385798644]  TranslationROffset=0  TranslationROffsetUnits=m  TranslationZOffset=0  TranslationZOffsetUnits=m  TranslationThetaOffset=0  TranslationThetaOffsetUnits=deg  RotationMethod=ArbitraryAxis  RotationAngleUnits=rad  RotationStandardAxis=+Z  RotationAngle=3.1415926535897896  RotationArbitraryAxis=[-1 5.1433426364519453e-33 -2.9461315815038046e-18]  FollAlignAxisA=+X  BaseAlignAxisA=+Y  FollAlignAxisB=+Y  BaseAlignAxisB=+Z  RotationMatrix=[1 0 0; 0 1 0; 0 0 1]  BlockFunction=simmechanics.library.frames_transforms.rigid_transform
      settings: SourceProductName=Simscape Multibody  SourceProductBaseCode=MS
  F : PMIOPort  Side=Left
  connections:
  ReferenceFrame/RConn1 -- Solid/RConn1 -- Transform/LConn1
  Transform/RConn1 -- F/RConn1

== matlab function Controlled Quadrotor2/Fix yaw angle ==
  data: yawangle input double; anglefix output double
function anglefix = fcn(yawangle)
%#codegen

if yawangle<0
    anglefix=2*pi-abs(yawangle);
else
    anglefix=yawangle;
end

== matlab function Controlled Quadrotor2/Position_Controller/calculate_desired_attitude ==
  data: accx_des input double; roll_des output double; accy_des input double; accz_des input double; yaw_des input double; pitch_des output double; tot_thrst_des output double
function [roll_des,pitch_des,tot_thrst_des] = fcn(accx_des,accy_des,accz_des,yaw_des)
%#codegen

%parameters
g=9.8;%m/s^2
m=(87+4*1.7)/1000;%Kg

roll_des= ( accx_des*sin(yaw_des) - accy_des*cos(yaw_des) )/g;
pitch_des= ( accx_des*cos(yaw_des) + accy_des*sin(yaw_des) )/g;
tot_thrst_des=m*accz_des;

% if roll_des<0
%     roll_des=2*pi-abs(roll_des);
% end

== matlab function Controlled Quadrotor1/Fix yaw angle ==
  data: yawangle input double; anglefix output double
function anglefix = fcn(yawangle)
%#codegen

if yawangle<0
    anglefix=2*pi-abs(yawangle);
else
    anglefix=yawangle;
end

== matlab function Controlled Quadrotor2/Quad and sensors/Ground Contact ==
  data: Alt input double; force output double; v input double; accz input double
function force = fcn(Alt,v,accz)
%#codegen

upper_bnd=200.0; % meters
lower_bnd=0; % meters
stiff_up=2e6; % N/m
stiff_low=2e6; % N/m
D_up= 150;% N/(m/s)
D_low=5; % N/(m/s)

%v=abs(v);
    if (Alt > upper_bnd)
        % Slider hits upper bound
        force = -1*(stiff_up * (Alt - upper_bnd) + D_up * v);
    elseif (Alt < lower_bnd)
        % Slider hits lower bound
        force = abs(stiff_low * (Alt - lower_bnd) + D_low * v);
        
        
    else
        % Slider is between hard stops
        force =0;
    end

== matlab function Controlled Quadrotor1/Position_Controller/calculate_desired_attitude ==
  data: accx_des input double; roll_des output double; accy_des input double; accz_des input double; yaw_des input double; pitch_des output double; tot_thrst_des output double
function [roll_des,pitch_des,tot_thrst_des] = fcn(accx_des,accy_des,accz_des,yaw_des)
%#codegen

%parameters
g=9.8;%m/s^2
m=(87+4*1.7)/1000;%Kg

roll_des= ( accx_des*sin(yaw_des) - accy_des*cos(yaw_des) )/g;
pitch_des= ( accx_des*cos(yaw_des) + accy_des*sin(yaw_des) )/g;
tot_thrst_des=m*accz_des;

% if roll_des<0
%     roll_des=2*pi-abs(roll_des);
% end

== matlab function Controlled Quadrotor1/Quad and sensors/Ground Contact ==
  data: Alt input double; force output double; v input double; accz input double
function force = fcn(Alt,v,accz)
%#codegen

upper_bnd=200.0; % meters
lower_bnd=0; % meters
stiff_up=2e6; % N/m
stiff_low=2e6; % N/m
D_up= 150;% N/(m/s)
D_low=5; % N/(m/s)

%v=abs(v);
    if (Alt > upper_bnd)
        % Slider hits upper bound
        force = -1*(stiff_up * (Alt - upper_bnd) + D_up * v);
    elseif (Alt < lower_bnd)
        % Slider hits lower bound
        force = abs(stiff_low * (Alt - lower_bnd) + D_low * v);
        
        
    else
        % Slider is between hard stops
        force =0;
    end
